simulink model "VehicleDynamicsSimulink"  (R2026a)
settings: Solver=ode45  StopTime=180  MinStep=0.005
InitFcn:
  | run('VehicleConfig.m')
libraries: eeGeneralControl x1, simulink_extras x1
settings Model: Creator=sh2323  LastModifiedBy=sh2323

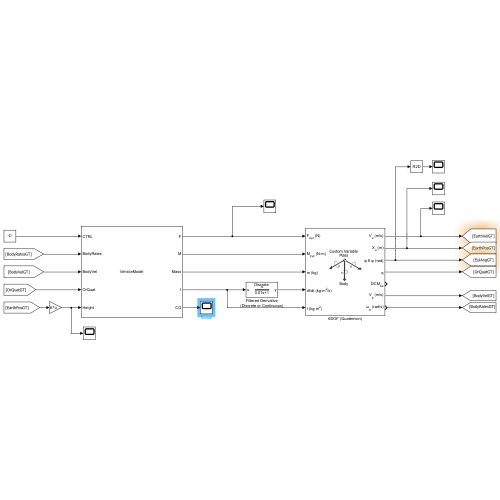
[thumbnail: Simulink's stored preview of the top-level diagram]
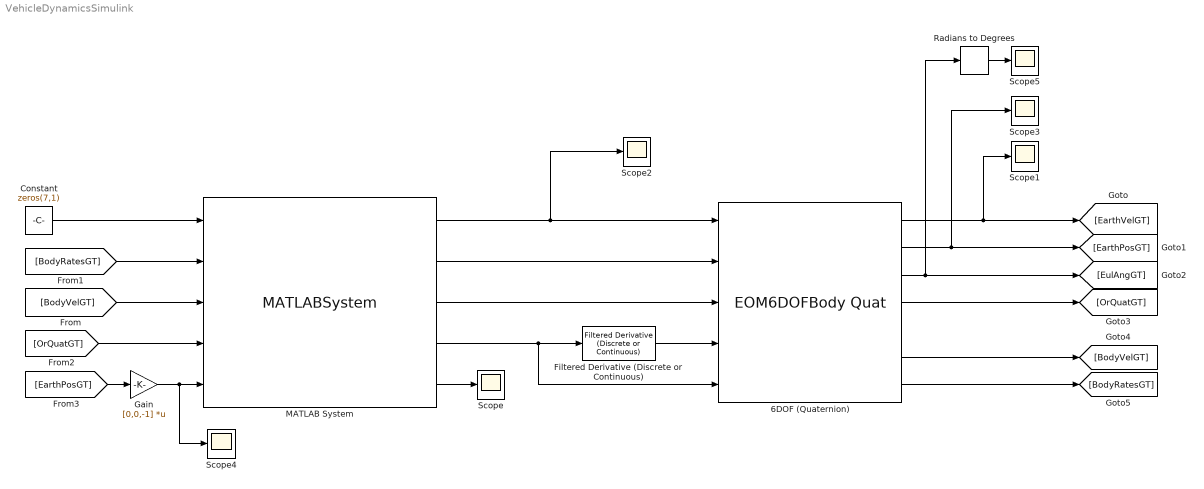
== system VehicleDynamicsSimulink ==
  6DOF (Quaternion) : EOM6DOFBodyQuat  mtype=Custom Variable  xme_0=[0 0 -500]  Vm_0=[20 0 0]
  Constant : Constant  Value=zeros(7,1)
  Filtered Derivative (Discrete or Continuous) : eeGeneralControl/Filtered Derivative (Discrete or Continuous)  K=1  T=0.01  B=inf  A=-inf  minRatio=10  init_option=Inherited from block input  x0=0  Ts=-1
      settings: LibrarySourceBlock=|
      | ee_sl_lib/General Control/Filtered Derivative
      | (Discrete or Continuous)
  Gain : Gain  Gain=[0,0,-1]  Multiplication=Matrix(K*u)
  MATLAB System : MATLABSystem  System=VehicleModel  Plane=plane  ModelName=ModelName  Rho=1.22  SimulateUsing=Interpreted execution
      mask Type: VehicleModel
  Radians to Degrees : simulink_extras/Transformations/Radians to Degrees
  Scope{,1..5} (6 alike) : Scope
      Scope settings: ActiveDisplayYMinimum=-0.18071321764401455  ActiveDisplayYMaximum=0.0200792464048905
      Scope1 settings: ActiveDisplayYMinimum=-1.9155713132710712  ActiveDisplayYMaximum=21.893952496252737
      Scope2 settings: ActiveDisplayYMinimum=-2620.3375888919372  ActiveDisplayYMaximum=306.23966868813  DataLoggingVariableName=ScopeData2
      Scope3 settings: ActiveDisplayYMinimum=-1  ActiveDisplayYMaximum=1  DataLoggingVariableName=ScopeData3
      Scope4 settings: ActiveDisplayYMinimum=-500.000387176247  ActiveDisplayYMaximum=-499.99926172234279  DataLoggingVariableName=ScopeData4
      Scope5 settings: ActiveDisplayYMinimum=-225  ActiveDisplayYMaximum=225  DataLoggingVariableName=ScopeData5
  wires:
  MATLAB System/1 -> Scope2/1, 6DOF (Quaternion)/1
  MATLAB System/2 -> 6DOF (Quaternion)/2
  MATLAB System/3 -> 6DOF (Quaternion)/3
  Filtered Derivative (Discrete or Continuous)/1 -> 6DOF (Quaternion)/4
  MATLAB System/4 -> 6DOF (Quaternion)/5, Filtered Derivative (Discrete or Continuous)/1
  MATLAB System/5 -> Scope/1
  6DOF (Quaternion)/1 -> Scope1/1, [EarthVelGT]
  6DOF (Quaternion)/2 -> Scope3/1, [EarthPosGT]
  6DOF (Quaternion)/3 -> Radians to Degrees/1, [EulAngGT]
  6DOF (Quaternion)/4 -> [OrQuatGT]
  6DOF (Quaternion)/6 -> [BodyVelGT]
  6DOF (Quaternion)/7 -> [BodyRatesGT]
  Constant/1 -> MATLAB System/1
  [BodyVelGT] -> MATLAB System/3
  [BodyRatesGT] -> MATLAB System/2
  [OrQuatGT] -> MATLAB System/4
  Gain/1 -> Scope4/1, MATLAB System/5
  [EarthPosGT] -> Gain/1
  Radians to Degrees/1 -> Scope5/1
